simulink model "LOPES_3D"  (R2015b)
settings: Solver=ode3  StartTime=0.0  StopTime=inf  FixedStep=ts  RelTol=1e-3
PostLoadFcn:
  | DataFileTemplate = 'd:\%d_LNMC_S01_SLRT_%i.mat';
InitFcn:
  | cd(fileparts(which(gcs)));
  | runScripts
StartFcn:
  | cd(fileparts(which(gcs)));
StopFcn:
  | SaveSLRTData(DataFileTemplate)
values from neighbouring files (symbols this model uses):
  SelectorLOPESInSize = 8    [setAnkleDepInd.m]
libraries: nmc x51, simulink x22, slrtlib x14, LopesDevelopmentLibrary x7, dspsigops x1
(part 1 of 2)
settings Model: xpc_rtwmakecfg_data=_xpciplib__xpcnblib__xpcetherlib__xpcether8255xlib__xpcetherGbElib_  SimulationMode=external  Creator=OortG  LastModifiedBy=brugtjh
settings SolverCC: EnableConcurrentExecution=on
settings DataIOCC: SaveFormat=Array
settings OptimizationCC: BlockReduction=off  OptimizeBlockIOStorage=off  BufferReuse=off  GlobalBufferReuse=off  ExpressionFolding=off  ExpressionDepthLimit=2147483647  LocalBlockOutputs=off
settings DebuggingCC: UnderspecifiedInitializationDetection=Classic  MergeDetectMultiDrivingBlocksExec=none  SolverPrmCheckMsg=warning  StateNameClashWarn=warning
settings HardwareCC: ProdBitPerPointer=32  ProdLargestAtomicFloat=None  ProdWordSize=32  ProdLongLongMode=on  ProdHWDeviceType=Generic->32-bit x86 compatible
settings RTWCC: SystemTargetFile=slrt.tlc  TLCOptions=-axPCMaxOverloads=999999 -axPCOverLoadLen=999999 -axPCStartupFlag=5  TemplateMakefile=slrt_default_tmf  Description=Simulink Real-Time
settings ConfigComp: CovModelRefEnable=Off

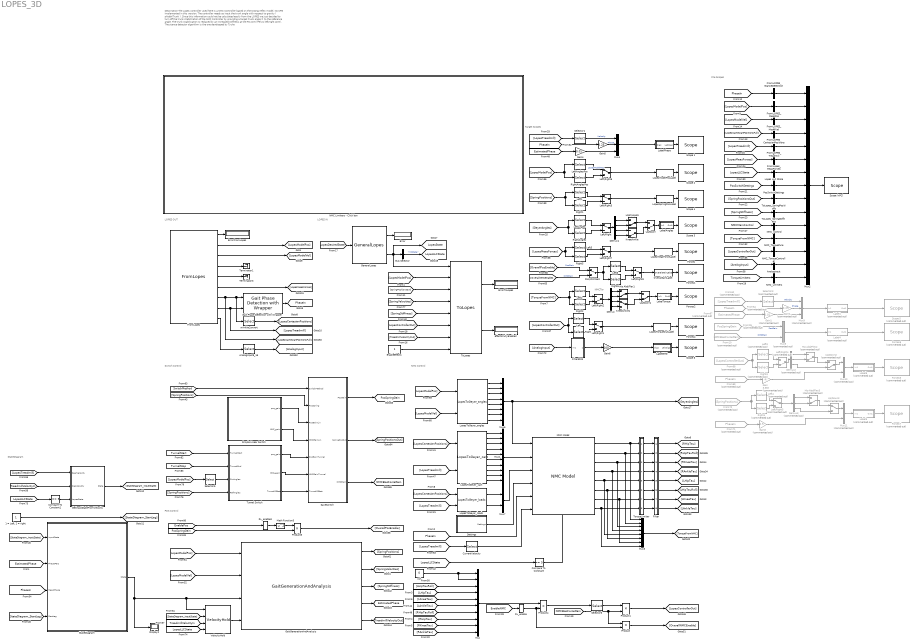
== system LOPES_3D ==
  note: File Scopes
  note: Description
      |
      | The Lopes controller used here is a NMC Controller based on the S.Song reflex model. No CPG Implemented in this version.
      |
      | The controller needs as input the trunk angle with respect to gravity ( phidphiTrunk ).
      | Since this information could not be calculated easily from the LOPES we just decided to turn off the trunk stabilization of the NMC Controller by providing a target trunk angle = to the reference angle.
      |
      | The trunk stabilization is replaced by an increased stiffness at the PZ joint (Pelvis left/right joint).
      |
      | The stance detector algorithm is the one developped by Tycho
  note: Target Scopes
  note: LOPES OUT
  note: LOPES IN
  note: NMC Control
  note: NMCTor
  note: Switch Control
  note: POS Control
  note: StateDiagram
  "1 = Left, 2 = right" : Constant
  AnalogInput : Concatenate  NumInputs=1
  AnalogInput9_16 : Selector  InputPortWidth=16  IndexOptions=Index vector (dialog)  Indices=9:16  OutputSizes=1
  Bus Selector : BusSelector  OutputSignals=llcState
  Compare To Constant : simulink/Logic and Bit Operations/Compare To Constant  relop===  const=5  OutDataTypeStr=boolean
  Compare To Constant1 : simulink/Logic and Bit Operations/Compare To Constant  relop===  const=5  OutDataTypeStr=boolean
  CurrentVelocity : Selector  InputPortWidth=7  IndexOptions=Index vector (dialog)  Indices=[2]  OutputSizes=1
  Demux : Demux
  Demux1 : Demux
  Demux2 : Demux  Commented=on  Outputs=3
  Demux3 : Demux  Commented=on  Outputs=3
  Display2 : Display
  EffectsFullyEnabled : Display
      settings: AttributesFormatString=%<Tag>
  EnableEffects : Constant  OutDataTypeStr=double
      settings: OpenFcn=|
      | b = get_param(gcb,'value');
      | if (strcmp(b,'1')),
      |   set_param (gcb,'value','0');
      | else
      |   set_param(gcb,'value','1');
      | end;
  Error : Display
      settings: AttributesFormatString=%<Tag>
  ErrorFromLopes : Display
      settings: AttributesFormatString=%<Tag>
  ErrorToLopes : Display
      settings: AttributesFormatString=%<Tag>
  Filter : Subsystem
  FilterEMG : Subsystem
  Forces : slrtlib/Displays and Logging/Scope   scopeno=6  scopetype=Target  autostart=on  viewmode=Graphical sliding  formatstr='%15.6f'  grid=on  ylimits=[0,0]  nosamples=5000  noprepostsamples=0  interleave=1  triggermode=FreeRun  triggersignal=1  trigsignalfromport=off  triggerlevel=0.0  triggerslope=Either  triggerscope=1  triggersample=0  filename=data.dat  mode=Lazy  writesize=512  autorestart=off  dynamicfilemode=off  maxwritefilesize=512*1024^2
  Forces1 : slrtlib/Displays and Logging/Scope   scopeno=7  scopetype=Target  autostart=on  viewmode=Graphical sliding  formatstr='%15.6f'  grid=on  ylimits=[0,0]  nosamples=5000  noprepostsamples=0  interleave=1  triggermode=FreeRun  triggersignal=1  trigsignalfromport=off  triggerlevel=0.0  triggerslope=Either  triggerscope=1  triggersample=0  filename=data.dat  mode=Lazy  writesize=512  autorestart=off  dynamicfilemode=off  maxwritefilesize=512*1024^2
  Forces2 : slrtlib/Displays and Logging/Scope   scopeno=8  scopetype=Target  autostart=on  viewmode=Graphical sliding  formatstr='%15.6f'  grid=on  ylimits=[0,0]  nosamples=5000  noprepostsamples=0  interleave=1  triggermode=FreeRun  triggersignal=1  trigsignalfromport=off  triggerlevel=0.0  triggerslope=Either  triggerscope=1  triggersample=0  filename=data.dat  mode=Lazy  writesize=512  autorestart=off  dynamicfilemode=off  maxwritefilesize=512*1024^2
  Forces4 : slrtlib/Displays and Logging/Scope   scopeno=9  scopetype=Target  autostart=on  viewmode=Graphical sliding  formatstr='%15.6f'  grid=on  ylimits=[0,0]  nosamples=5000  noprepostsamples=0  interleave=1  triggermode=FreeRun  triggersignal=1  trigsignalfromport=off  triggerlevel=0.0  triggerslope=Either  triggerscope=1  triggersample=0  filename=data.dat  mode=Lazy  writesize=512  autorestart=off  dynamicfilemode=off  maxwritefilesize=512*1024^2
  Forces5 : slrtlib/Displays and Logging/Scope   Commented=on  scopeno=33  scopetype=Target  autostart=on  viewmode=Graphical sliding  formatstr='%15.6f'  grid=on  ylimits=[-20,20]  nosamples=5000  noprepostsamples=0  interleave=1  triggermode=FreeRun  triggersignal=1  trigsignalfromport=off  triggerlevel=0.0  triggerslope=Either  triggerscope=1  triggersample=0  filename=data.dat  mode=Lazy  writesize=512  autorestart=off  dynamicfilemode=off  maxwritefilesize=512*1024^2
  Forces6 : slrtlib/Displays and Logging/Scope   Commented=on  scopeno=22  scopetype=Target  autostart=on  viewmode=Graphical sliding  formatstr='%15.6f'  grid=on  ylimits=[0,0]  nosamples=5000  noprepostsamples=0  interleave=1  triggermode=FreeRun  triggersignal=1  trigsignalfromport=off  triggerlevel=0.0  triggerslope=Either  triggerscope=1  triggersample=0  filename=data.dat  mode=Lazy  writesize=512  autorestart=off  dynamicfilemode=off  maxwritefilesize=512*1024^2
  Forces7 : slrtlib/Displays and Logging/Scope   Commented=on  scopeno=44  scopetype=Target  autostart=on  viewmode=Graphical sliding  formatstr='%15.6f'  grid=on  ylimits=[-3,3]  nosamples=5000  noprepostsamples=0  interleave=1  triggermode=FreeRun  triggersignal=1  trigsignalfromport=off  triggerlevel=0.0  triggerslope=Either  triggerscope=1  triggersample=0  filename=data.dat  mode=Lazy  writesize=512  autorestart=off  dynamicfilemode=off  maxwritefilesize=512*1024^2
  From10 : From  Commented=on  GotoTag=NMCBiasForceGain  TagVisibility=global
  From26 : From  Commented=on  GotoTag=PosSpringGain  TagVisibility=global
  From62 : From  Commented=on  GotoTag=LopesTreadmill
  From64 : From  Commented=on  GotoTag=PhaseIn  TagVisibility=global
  From67 : From  Commented=on  GotoTag=EstimatedPhase  TagVisibility=global
  From68 : From  Commented=on  GotoTag=LopesControllerOut
  From69 : From  Commented=on  GotoTag=PhaseIn  TagVisibility=global
  From70 : From  Commented=on  GotoTag=SpringPositions
  From71 : From  Commented=on  GotoTag=PhaseIn  TagVisibility=global
  FromLOPES_CartesianPositions : Concatenate  NumInputs=1
  FromLOPES_MeasPos : Concatenate  NumInputs=1
  FromLOPES_ModelVel : Concatenate  NumInputs=1
  FromLOPES_StanceDetection : Concatenate  NumInputs=1
  FromLOPES_Treadmill : Concatenate  NumInputs=1
  FromLopes : LopesDevelopmentLibrary/Robot control blocks/FromLopes
  FromLopes_MeasForces : Concatenate  NumInputs=1
  Gain : Gain  Commented=on  Gain=3.333
  Gain1 : Gain  Commented=on  Gain=0.01
  Gain2 : Gain  Commented=on  Gain=0.25
  Gain3 : Gain  Commented=on  Gain=0.5
  Gain4 : Gain  Gain=0.01
  Gain5 : Gain  Gain=0.25
  Gain6 : Gain  Gain=100
  Gait Phase Detection with Wrapper : LopesDevelopmentLibrary/GaitPhaseDetection/Gait Phase Detection with Wrapper
  GaitGenerationAndAnalysis : LopesDevelopmentLibrary/GaitGenerationExtra/GaitGenerationAndAnalysis
      link override "CalculateBreaksCoefs/Calculate/StartLeft ": SetVelocity=0.1
      link override CalculateBreaksCoefs/Calculate/StartRight: SetVelocity=0.1
      link override CalculateBreaksCoefs/Calculate/StopLeft: SetVelocity=0.3
      link override CalculateBreaksCoefs/Calculate/StopRight: SetVelocity=0.3
      link override PhaseEstimatorAoyagi_wPI_Extra: AoyagiFilterGain=2
  GeneralLopes : LopesDevelopmentLibrary/Robot control blocks/GeneralLopes
  GetInputStateFromVelocity : Subsystem
  Hip Abd/Flex1 : ManualSwitch  CurrentSetting=0
  Hip Abd/Flex2 : ManualSwitch  Commented=on  CurrentSetting=0
  Hip Abd/Flex3 : ManualSwitch  Commented=on  CurrentSetting=0
  HipFl/HipAb : ManualSwitch  CurrentSetting=0
  Knee/Ankle : ManualSwitch  CurrentSetting=0
  Knee/Ankle1 : ManualSwitch
  Label1 : Subsystem  Commented=on
  Label4 : Subsystem  Commented=on
  Label5 : Subsystem  Commented=on
  Label6 : Subsystem  Commented=on
  LabelAngles : Subsystem
  LabelEMG : Subsystem
  LabelPhase : Subsystem
  LabelTorque : Subsystem
  Left{,1,5..6} (4 alike) : Selector  InputPortWidth=SelectorScopesSize  IndexOptions=Index vector (dialog)  Indices=SelectorScopesLeft  OutputSizes=1
  Left/Right{,1,3,6..7} (5 alike) : ManualSwitch
  Left/Right2 : ManualSwitch  CurrentSetting=0
  Left/Right4 : ManualSwitch  Commented=on  CurrentSetting=0
  Left/Right5 : ManualSwitch  Commented=on
  "Left/Right8 " : ManualSwitch
  Left2 : Selector  InputPortWidth=8  IndexOptions=Index vector (dialog)  Indices=[5,6,7,8]  OutputSizes=1
  Left3 : Selector  Commented=on  InputPortWidth=SelectorScopesSize  IndexOptions=Index vector (dialog)  Indices=SelectorScopesLeft  OutputSizes=1
  Left4 : Selector  Commented=on  InputPortWidth=SelectorScopesSize  IndexOptions=Index vector (dialog)  Indices=SelectorScopesLeft  OutputSizes=1
  LeftAngles : Selector  InputPortWidth=16  IndexOptions=Index vector (dialog)  Indices=[1,3,5,7]  OutputSizes=1
  LeftAnglesPos : Selector  InputPortWidth=SelectorLOPESModelPosSize  IndexOptions=Index vector (dialog)  Indices=SelectorScopesLeft  OutputSizes=1
  Lopes LLC State : Concatenate  NumInputs=1
  LopesMeasForceLabel : nmc/LopesMeasForceLabel
  LopesModelPosLabel : nmc/LopesModelPosLabel
  LopesSpringPosLabel : nmc/LopesSpringPosLabel
  LopesToGeyer_angles : nmc/LopesToGeyer_angles
  LopesToGeyer_cart : nmc/LopesToGeyer_cart
  LopesToGeyer_loads : nmc/LopesToGeyer_loads
  LopesTorqueOutLabel : nmc/LopesTorqueOutLabel
  Math Function3 : Math  Operator=square  SaturateOnIntegerOverflow=on
  Mux : Mux  Inputs=10
  Mux1 : Mux  Inputs=10
  Mux10 : Mux  Commented=on  Inputs=2
  Mux11 : Mux  Commented=on  Inputs=2
  Mux2 : Mux  Inputs=15
  Mux3 : Mux  Inputs=8
  Mux4 : Mux  Inputs=3
  Mux5 : Mux  Commented=on  Inputs=2
  Mux6 : Mux  Inputs=8
  Mux7 : Mux  Inputs=2
  Mux9 : Mux  Commented=on  Inputs=3
  NMC Limiters - Click box : Subsystem  mask{LopesDesiredState=Init, VelocityTreadmill=1, PercLimiterRate=20, InfoShow_LLC=0, InfoShow_Blue=1, InfoShow_Init=0, InfoShow_Motors=0, InfoShow_Treadmill=0, InfoShow_Patient=1, EnablePos=Enable, PosControlType=Linear, PosLimiterPercentageSymmetric=0.0, PosLimiterPercentagePelvis=0.0, PosLimiterPercentageLeft=8.0, PosLimiterPercentageRight=0.0, DisableAddPelvis=off, DisableAddLeft=off, DisableAddRight=off, Pos_Tunnel_PelvisX=0.010, Pos_Tunnel_PelvisZ=0.010, Pos_Tunnel_HipAdd=0.100, Pos_Tunnel_PelvisX_Out=0.020, Pos_Tunnel_PelvisZ_Out=0.020, Pos_Tunnel_HipAdd_Out=0.200, Pos_Tunnel_HipFlx=0.100, Pos_Tunnel_Knee=0.100, Pos_Tunnel_Ankle=0.200, Pos_Tunnel_HipFlx_Out=0.200, Pos_Tunnel_Knee_Out=0.200, Pos_Tunnel_Ankle_Out=0.400, EnableNMC=Enable, TorqueLimiterPercentageSymmetric=0, TorqueLimiterPercentageLeft=0, TorqueLimiterPercentageRight=0, GradientFunctionSwitch=Per Gradient, NMC_HipAddAbd_Percentage=100.0, NMC_HipFlexExt_Percentage=100, NMC_KneeFlexExt_Percentage=0, NMC_AnkleDorsPlant_Percentage=0, NMC_HipAdd_Percentage=100.0, NMC_HipAbd_Percentage=100.0, NMC_HipFlexors_Percentage=100, NMC_HipExtensors_Percentage=100, NMC_KneeFlexors_Percentage=0, NMC_KneeExtensors_Percentage=100, NMC_AnkleDFlexor_Percentage=0, NMC_AnklePFlexors_Percentage=0, NMC_HipMuscles_AbAd_Percentage=100.0, NMC_HipMuscles_FE_Percentage=100.0, NMC_BiArticularMuscles_HK_Percentage=100.0, NMC_KneeMuscles_Percentage=100.0, NMC_BiArticularMuscles_KA_Percentage=0.0, NMC_AnkleMuscles_Percentage=0.0, EnableJointLimits=Disable, UseConstantPitch=Enable, UsePredictedAnkle=Enable, KneeAngleBias=0, FilterFreq=25, EnableStandingStill=Enable, StandingStillLimitFront=0.10, StandingStillLimitSide=0.20}
      mask prompts: LopesDesiredState "Lopes State (Desired):"; VelocityTreadmill "Treadmill Velocity (m/s):"; PercLimiterRate "Limiter Rate (%/s):"; InfoShow_LLC "LLC State"; InfoShow_Blue "Blue Cabinet Pressed"; InfoShow_Init "Init OK"; InfoShow_Motors "Motors OK"; InfoShow_Treadmill "Treadmill Empty"; InfoShow_Patient "PatientDefined"; EnablePos "Enable/Disable Pos"; PosLimiterPercentageSymmetric "Overal Gain:"; PosLimiterPercentagePelvis "Pelvis Gain:"; PosLimiterPercentageLeft "Left Gain:"; PosLimiterPercentageRight "Right Gain:"; DisableAddPelvis "Disable Tunnel Pelvis"; DisableAddLeft "Disable Tunnel Left"; DisableAddRight "Disable Tunnel Right"; Pos_Tunnel_PelvisX "Pelvis (x) (m):"; Pos_Tunnel_PelvisZ "Pelvis (z) (m):"; Pos_Tunnel_HipAdd "Hip Add/Abd (rad):"; Pos_Tunnel_PelvisX_Out "Pelvis (x) (m):"; Pos_Tunnel_PelvisZ_Out "Pelvis (z) (m):"; Pos_Tunnel_HipAdd_Out "Hip Add/Abd (rad):"; Pos_Tunnel_HipFlx "Hip Flx/Ext (rad):"; Pos_Tunnel_Knee "Knee Flx/Ext (rad):"; Pos_Tunnel_Ankle "Ankle Flx/Ext (rad):"; Pos_Tunnel_HipFlx_Out "Hip Flx/Ext (rad):"; Pos_Tunnel_Knee_Out "Knee Flx/Ext (rad):"; Pos_Tunnel_Ankle_Out "Ankle Flx/Ext (rad):"; EnableNMC "Enable/Disable NMC"; TorqueLimiterPercentageSymmetric "Overal Gain:"; TorqueLimiterPercentageLeft "Left Gain:"; TorqueLimiterPercentageRight "Right Gain:"; NMC_HipAddAbd_Percentage "Hip Add/Abd Percentage"; NMC_HipFlexExt_Percentage "Hip Flex/Ext Percentage"; NMC_KneeFlexExt_Percentage "Knee Flex/Ext Percentage"; NMC_AnkleDorsPlant_Percentage "Ankle Dorsi/Plantar Percentage"; NMC_HipAdd_Percentage "Hip Adduction Percentage"; NMC_HipAbd_Percentage "Hip Abduction Percentage"; NMC_HipFlexors_Percentage "Hip Flexor Percentage"; NMC_HipExtensors_Percentage "Hip Extensor Percentage"; NMC_KneeFlexors_Percentage "Knee Flexor Percentage"; NMC_KneeExtensors_Percentage "Knee Extensor Percentage"; NMC_AnkleDFlexor_Percentage "Ankle DorsiFlexor Percentage"; NMC_AnklePFlexors_Percentage "Ankle PlantarFlexor Percentage"; NMC_HipMuscles_AbAd_Percentage "Hip (Mono) (Abd/Add)"; NMC_HipMuscles_FE_Percentage "Hip (Mono) (Flex./Ext.)"; NMC_BiArticularMuscles_HK_Percentage "Hip/Knee (BiArt)"; NMC_KneeMuscles_Percentage "Knee (Mono)"; NMC_BiArticularMuscles_KA_Percentage "Knee/Ankle (BiArt)"; NMC_AnkleMuscles_Percentage "Ankle Muscles"; EnableJointLimits "Enable/Disable Joint Limits"; UseConstantPitch "Enable/Disable Constant Pitch"; UsePredictedAnkle "Enable/Disable Predicted Ankle"; KneeAngleBias "Knee Angle Bias (Rad):"; FilterFreq "Filter Frequency (Hz):"; EnableStandingStill "Enable/Disable Standing Still"; StandingStillLimitFront "Front Velocity Limit"; StandingStillLimitSide "Side Velocity Limit"
      mask TypeOptions LopesDesiredState: Off | Init | Force
      mask Callback LopesDesiredState:
      | button_value = get_param(gcb,'LopesDesiredState');
      | 
      | if strcmp(button_value,'Off')
      |      set_param([gcb '/DesiredState'],'Value',num2str(0));
      | elseif strcmp(button_value,'Init')
      |     set_param([gcb '/DesiredState'],'Value',num2str(1));
      | elseif strcmp(button_value,'Force')
      |     set_param([gcb '/DesiredState'],'Value',num2str(5));
      | end
      mask Callback PercLimiterRate:
      | button_value = get_param(gcb,'PercLimiterRate');
      | set_param([gcb '/PercLimiterRate'],'Value',num2str(button_value));
      mask TypeOptions EnablePos: Enable | Disable
      mask Callback EnablePos:
      | button_value = get_param(gcb,'EnablePos');
      | 
      | if strcmp(button_value,'Enable')
      |      set_param([gcb '/EnablePos'],'Value',num2str(1));
      |      set_param([gcb '/DisableAddAll'],'Value','0');
      | else
      |     set_param([gcb '/EnablePos'],'Value',num2str(0));
      |     set_param([gcb '/DisableAddAll'],'Value','2*pi');
      | end
      mask TypeOptions PosControlType: Linear | Tunnel
      mask Callback PosControlType:
      | button_value = get_param(gcb,'PosControlType');
      | 
      | maskHandle = Simulink.Mask.get(gcb);
      | buttonHandleTunnel1 = maskHandle.getDialogControl('ContainerTunnel1');
      | buttonHandleTunnel2 = maskHandle.getDialogControl('ContainerTunnel2');
      | % buttonHandleDisableTunnelPelvis = maskHandle.getParameter('DisableAddPelvis');
      | % buttonHandleDisableTunnelLeft = maskHandle.getParameter('DisableAddLeft');
      | % buttonHandleDisableTunnelRight = maskHandle.getParameter('DisableAddRight');
      | if strcmp(button_value,'Tunnel')
      |     set_param([gcb '/PosControlType'],'Value',num2str(1));
      |     buttonHandleTunnel1.Enabled = 'on';
      |     buttonHandleTunnel2.Enabled = 'on';
      | %     buttonHandleDisableTunnelPelvis.Enabled = 'on';
      | %     buttonHandleDisableTunnelLeft.Enabled = 'on';
      | %     buttonHandleDisableTunnelRight.Enabled = 'on';
      | else
      |     set_param([gcb '/PosControlType'],'Value',num2str(0));
      |     buttonHandleTunnel1.Enabled = 'off';
      |     buttonHandleTunnel2.Enabled = 'off';
      | %     buttonHandleDisableTunnelPelvis.Enabled = 'off';
      | %     buttonHandleDisableTunnelLeft.Enabled = 'off';
      | %     buttonHandleDisableTunnelRight.Enabled = 'off';
      | end
      mask Callback PosLimiterPercentageSymmetric:
      | %% Overal Gain
      | value_new = get_param(gcb,'PosLimiterPercentageSymmetric');
      | value = get_param([gcb,'/PosLimiterPercentage'],'Value');
      | 
      | if ~strcmp(value,value_new)
      | % Also setting other sliders
      | set_param(gcb,'PosLimiterPercentagePelvis',value_new);
      | set_param(gcb,'PosLimiterPercentageLeft',value_new);
      | set_param(gcb,'PosLimiterPercentageRight',value_new);
      | 
      | % Setting Overal Slider (Only used for logging)
      | set_param([gcb '/PosLimiterPercentage'],'Value',value_new);
      | end
      mask Callback DisableAddPelvis:
      | value = get_param(gcb,'DisableAddPelvis');
      | 
      | if strcmp(value,'on')
      |     set_param([gcb,'/DisableAddPelvis'],'Value','2*pi')
      | else
      | set_param([gcb,'/DisableAddPelvis'],'Value','0')
      | end
      mask Callback DisableAddLeft:
      | value = get_param(gcb,'DisableAddLeft');
      | 
      | if strcmp(value,'on')
      |     set_param([gcb,'/DisableAddLeft'],'Value','2*pi')
      | else
      | set_param([gcb,'/DisableAddLeft'],'Value','0')
      | end
      mask Callback DisableAddRight:
      | value = get_param(gcb,'DisableAddRight');
      | 
      | if strcmp(value,'on')
      |     set_param([gcb,'/DisableAddRight'],'Value','2*pi')
      | else
      |     set_param([gcb,'/DisableAddRight'],'Value','0')
      | end
      mask Callback Pos_Tunnel_PelvisX:
      | %% Overal Gain
      | value_first = get_param(gcb,'Pos_Tunnel_PelvisX');
      | value = get_param(gcb,'Pos_Tunnel_PelvisX_Out');
      | 
      | if str2num(value) < str2num(value_first)
      |     set_param(gcb,'Pos_Tunnel_PelvisX_Out',value_first);
      | end
      mask Callback Pos_Tunnel_PelvisZ:
      | %% Overal Gain
      | value_first = get_param(gcb,'Pos_Tunnel_PelvisZ');
      | value = get_param(gcb,'Pos_Tunnel_PelvisZ_Out');
      | 
      | if str2num(value) < str2num(value_first)
      |     set_param(gcb,'Pos_Tunnel_PelvisZ_Out',value_first);
      | end
      mask Callback Pos_Tunnel_HipAdd:
      | %% Overal Gain
      | value_first = get_param(gcb,'Pos_Tunnel_HipAdd');
      | value = get_param(gcb,'Pos_Tunnel_HipAdd_Out');
      | 
      | if str2num(value) < str2num(value_first)
      |     set_param(gcb,'Pos_Tunnel_HipAdd_Out',value_first);
      | end
      mask Callback Pos_Tunnel_PelvisX_Out:
      | %% Overal Gain
      | value = get_param(gcb,'Pos_Tunnel_PelvisX_Out');
      | value_first = get_param(gcb,'Pos_Tunnel_PelvisX');
      | 
      | if str2num(value) < str2num(value_first)
      |     set_param(gcb,'Pos_Tunnel_PelvisX_Out',value_first);
      | end
      mask Callback Pos_Tunnel_PelvisZ_Out:
      | %% Overal Gain
      | value = get_param(gcb,'Pos_Tunnel_PelvisZ_Out');
      | value_first = get_param(gcb,'Pos_Tunnel_PelvisZ');
      | 
      | if str2num(value) < str2num(value_first)
      |     set_param(gcb,'Pos_Tunnel_PelvisZ_Out',value_first);
      | end
      mask Callback Pos_Tunnel_HipAdd_Out:
      | %% Overal Gain
      | value = get_param(gcb,'Pos_Tunnel_HipAdd_Out');
      | value_first = get_param(gcb,'Pos_Tunnel_HipAdd');
      | 
      | if str2num(value) < str2num(value_first)
      |     set_param(gcb,'Pos_Tunnel_HipAdd_Out',value_first);
      | end
      mask Callback Pos_Tunnel_HipFlx:
      | %% Overal Gain
      | value_first = get_param(gcb,'Pos_Tunnel_HipFlx');
      | value = get_param(gcb,'Pos_Tunnel_HipFlx_Out');
      | 
      | if str2num(value) < str2num(value_first)
      |     set_param(gcb,'Pos_Tunnel_HipFlx_Out',value_first);
      | end
      mask Callback Pos_Tunnel_Knee:
      | %% Overal Gain
      | value_first = get_param(gcb,'Pos_Tunnel_Knee');
      | value = get_param(gcb,'Pos_Tunnel_Knee_Out');
      | 
      | if str2num(value) < str2num(value_first)
      |     set_param(gcb,'Pos_Tunnel_Knee_Out',value_first);
      | end
      mask Callback Pos_Tunnel_Ankle:
      | %% Overal Gain
      | value_first = get_param(gcb,'Pos_Tunnel_Ankle');
      | value = get_param(gcb,'Pos_Tunnel_Ankle_Out');
      | 
      | if str2num(value) < str2num(value_first)
      |     set_param(gcb,'Pos_Tunnel_Ankle_Out',value_first);
      | end
      mask Callback Pos_Tunnel_HipFlx_Out:
      | %% Overal Gain
      | value = get_param(gcb,'Pos_Tunnel_HipFlx_Out');
      | value_first = get_param(gcb,'Pos_Tunnel_HipFlx');
      | 
      | if str2num(value) < str2num(value_first)
      |     set_param(gcb,'Pos_Tunnel_HipFlx_Out',value_first);
      | end
      mask Callback Pos_Tunnel_Knee_Out:
      | %% Overal Gain
      | value = get_param(gcb,'Pos_Tunnel_Knee_Out');
      | value_first = get_param(gcb,'Pos_Tunnel_Knee');
      | 
      | if str2num(value) < str2num(value_first)
      |     set_param(gcb,'Pos_Tunnel_Knee_Out',value_first);
      | end
      mask Callback Pos_Tunnel_Ankle_Out:
      | %% Overal Gain
      | value = get_param(gcb,'Pos_Tunnel_Ankle_Out');
      | value_first = get_param(gcb,'Pos_Tunnel_Ankle');
      | 
      | if str2num(value) < str2num(value_first)
      |     set_param(gcb,'Pos_Tunnel_Ankle_Out',value_first);
      | end
      mask TypeOptions EnableNMC: Enable | Disable
      mask Callback EnableNMC:
      | button_value = get_param(gcb,'EnableNMC');
      | 
      | if strcmp(button_value,'Enable')
      |      set_param([gcb '/EnableNMC'],'Value',num2str(1));
      | else
      |     set_param([gcb '/EnableNMC'],'Value',num2str(0));
      | end
      mask Callback TorqueLimiterPercentageSymmetric:
      | %% Overal Gain
      | value_new = get_param(gcb,'TorqueLimiterPercentageSymmetric');
      | value = get_param([gcb,'/TorqueLimiterPercentageSymmetric'],'Value');
      | 
      | if ~strcmp(value,value_new)
      | % Also setting other sliders
      | set_param(gcb,'TorqueLimiterPercentageLeft',value_new);
      | set_param(gcb,'TorqueLimiterPercentageRight',value_new);
      | 
      | % Setting Overal Slider (Only used for logging)
      | set_param([gcb '/TorqueLimiterPercentageSymmetric'],'Value',value_new);
      | end
      mask TypeOptions GradientFunctionSwitch: Per Joint | Per Function | Per Gradient
      mask Callback GradientFunctionSwitch:
      | blk = gcb;
      | button_value = get_param(gcb,'GradientFunctionSwitch');
      | 
      | if strcmp(button_value,'Per Joint')
      |     DesiredControlMethod = 1;
      | elseif strcmp(button_value,'Per Function')
      |     DesiredControlMethod = 2;
      | elseif strcmp(button_value,'Per Gradient')
      |     DesiredControlMethod = 3;
      | end
      | 
      | set_param([gcb '/LimiterMethod'],'Value',num2str(DesiredControlMethod));
      | 
      | %% Disabling one or the other
      | maskHandle = Simulink.Mask.get(gcb);
      | buttonHandleGradient = maskHandle.getDialogControl('Container_Gradient');
      | buttonHandleFunction = maskHandle.getDialogControl('Container_Function');
      | buttonHandleJoint = maskHandle.getDialogControl('Container_Joint');
      | if DesiredControlMethod == 1 %Per Joint
      |     buttonHandleGradient.Enabled = 'off';
      |     buttonHandleFunction.Enabled = 'off';
      |     buttonHandleJoint.Enabled = 'on';
      | elseif DesiredControlMethod == 2 %Per Function
      |     buttonHandleGradient.Enabled = 'off';
      |     buttonHandleFunction.Enabled = 'on';
      |     buttonHandleJoint.Enabled = 'off';
      | elseif DesiredControlMethod == 3 %Per Gradient
      |     buttonHandleGradient.Enabled = 'on';
      |     buttonHandleFunction.Enabled = 'off';
      |     buttonHandleJoint.Enabled = 'off';
      | end
      mask Callback NMC_HipAddAbd_Percentage:
      | %Setting values hip add/abd
      | if str2num(get_param([gcb '/LimiterMethod'],'Value')) == 1;
      |     %Also setting values of sliders per joint/per location
      |     set_param(gcb,'NMC_HipAdd_Percentage',get_param(gcb,'NMC_HipAddAbd_Percentage'))
      |     set_param(gcb,'NMC_HipAbd_Percentage',get_param(gcb,'NMC_HipAddAbd_Percentage'))
      |     set_param(gcb,'NMC_HipMuscles_AbAd_Percentage',get_param(gcb,'NMC_HipAddAbd_Percentage'))
      | end
      mask Callback NMC_HipFlexExt_Percentage:
      | if str2num(get_param([gcb '/LimiterMethod'],'Value')) == 1;
      | %Also setting values of sliders per function/per location
      | %Per Function
      | set_param(gcb,'NMC_HipFlexors_Percentage',str2num(get_param(gcb,'NMC_HipFlexExt_Percentage')))
      | set_param(gcb,'NMC_HipExtensors_Percentage',str2num(get_param(gcb,'NMC_HipFlexExt_Percentage')))
      | 
      | %Per Location
      | set_param(gcb,'NMC_HipMuscles_FE_Percentage',str2num(get_param(gcb,'NMC_HipFlexExt_Percentage')))
      | set_param(gcb,'NMC_BiArticularMuscles_HK_Percentage',min([str2num(get_param(gcb,'NMC_HipFlexExt_Percentage')) str2num(get_param(gcb,'NMC_KneeFlexExt_Percentage'))]))
      | end
      mask Callback NMC_KneeFlexExt_Percentage:
      | if str2num(get_param([gcb '/LimiterMethod'],'Value')) == 1;
      | %Also setting values of sliders per joint/per location
      | set_param(gcb,'NMC_KneeFlexors_Percentage',str2num(get_param(gcb,'NMC_KneeFlexExt_Percentage')))
      | set_param(gcb,'NMC_KneeExtensors_Percentage',str2num(get_param(gcb,'NMC_KneeFlexExt_Percentage')))
      | set_param(gcb,'NMC_KneeMuscles_Percentage',str2num(get_param(gcb,'NMC_KneeFlexExt_Percentage')))
      | set_param(gcb,'NMC_BiArticularMuscles_KA_Percentage',min([str2num(get_param(gcb,'NMC_KneeFlexExt_Percentage')) str2num(get_param(gcb,'NMC_AnkleDorsPlant_Percentage'))]))
      | set_param(gcb,'NMC_BiArticularMuscles_HK_Percentage',min([str2num(get_param(gcb,'NMC_HipFlexExt_Percentage')) str2num(get_param(gcb,'NMC_KneeFlexExt_Percentage'))]))
      | end
      mask Callback NMC_AnkleDorsPlant_Percentage:
      | if str2num(get_param([gcb '/LimiterMethod'],'Value')) == 1;
      | %Also setting values of sliders per joint/per location
      | set_param(gcb,'NMC_AnkleDFlexor_Percentage',str2num(get_param(gcb,'NMC_AnkleDorsPlant_Percentage')))
      | set_param(gcb,'NMC_AnklePFlexors_Percentage',str2num(get_param(gcb,'NMC_AnkleDorsPlant_Percentage')))
      | set_param(gcb,'NMC_AnkleMuscles_Percentage',str2num(get_param(gcb,'NMC_AnkleDorsPlant_Percentage')))
      | set_param(gcb,'NMC_BiArticularMuscles_KA_Percentage',min([str2num(get_param(gcb,'NMC_KneeFlexExt_Percentage')) str2num(get_param(gcb,'NMC_AnkleDorsPlant_Percentage'))]))
      | end
      mask Callback NMC_HipAdd_Percentage:
      | if str2num(get_param([gcb '/LimiterMethod'],'Value')) == 2;
      | %Also setting values of sliders per joint/per location
      | set_param(gcb,'NMC_HipAddAbd_Percentage',min([str2num(get_param(gcb,'NMC_HipAdd_Percentage')) str2num(get_param(gcb,'NMC_HipAbd_Percentage'))]))
      | set_param(gcb,'NMC_HipMuscles_AbAd_Percentage',min([str2num(get_param(gcb,'NMC_HipAdd_Percentage')) str2num(get_param(gcb,'NMC_HipAbd_Percentage'))]))
      | end
      mask Callback NMC_HipAbd_Percentage:
      | if str2num(get_param([gcb '/LimiterMethod'],'Value')) == 2;
      | %Also setting values of sliders per joint/per location
      | set_param(gcb,'NMC_HipAddAbd_Percentage',min([str2num(get_param(gcb,'NMC_HipAdd_Percentage')) str2num(get_param(gcb,'NMC_HipAbd_Percentage'))]))
      | set_param(gcb,'NMC_HipMuscles_AbAd_Percentage',min([str2num(get_param(gcb,'NMC_HipAdd_Percentage')) str2num(get_param(gcb,'NMC_HipAbd_Percentage'))]))
      | end
      mask Callback NMC_HipFlexors_Percentage:
      | if str2num(get_param([gcb '/LimiterMethod'],'Value')) == 2;
      | 
      | %% Also setting values of sliders per joint/per location
      | % Per Joint
      | set_param(gcb,'NMC_HipFlexExt_Percentage',min([str2num(get_param(gcb,'NMC_HipFlexors_Percentage')) str2num(get_param(gcb,'NMC_HipExtensors_Percentage'))]))
      | 
      | % Per Location
      | set_param(gcb,'NMC_HipMuscles_FE_Percentage',min([str2num(get_param(gcb,'NMC_HipFlexors_Percentage')) str2num(get_param(gcb,'NMC_HipExtensors_Percentage'))]))
      | set_param(gcb,'NMC_BiArticularMuscles_HK_Percentage',min([str2num(get_param(gcb,'NMC_KneeExtensors_Percentage')) str2num(get_param(gcb,'NMC_KneeFlexors_Percentage')) str2num(get_param(gcb,'NMC_HipFlexors_Percentage')) str2num(get_param(gcb,'NMC_HipExtensors_Percentage'))]))
      | end
      mask Callback NMC_HipExtensors_Percentage:
      | if str2num(get_param([gcb '/LimiterMethod'],'Value')) == 2;
      | %Also setting values of sliders per joint/per location
      | set_param(gcb,'NMC_HipFlexExt_Percentage',min([str2num(get_param(gcb,'NMC_HipFlexors_Percentage')) str2num(get_param(gcb,'NMC_HipExtensors_Percentage'))]))
      | set_param(gcb,'NMC_HipMuscles_FE_Percentage',min([str2num(get_param(gcb,'NMC_HipFlexors_Percentage')) str2num(get_param(gcb,'NMC_HipExtensors_Percentage'))]))
      | set_param(gcb,'NMC_BiArticularMuscles_HK_Percentage',min([str2num(get_param(gcb,'NMC_KneeExtensors_Percentage')) str2num(get_param(gcb,'NMC_KneeFlexors_Percentage')) str2num(get_param(gcb,'NMC_HipFlexors_Percentage')) str2num(get_param(gcb,'NMC_HipExtensors_Percentage'))]))
      | end
      mask Callback NMC_KneeFlexors_Percentage:
      | if str2num(get_param([gcb '/LimiterMethod'],'Value')) == 2;
      | %Also setting values of sliders per joint/per location
      | set_param(gcb,'NMC_KneeFlexExt_Percentage',min([str2num(get_param(gcb,'NMC_KneeExtensors_Percentage')) str2num(get_param(gcb,'NMC_KneeFlexors_Percentage'))]))
      | set_param(gcb,'NMC_KneeMuscles_Percentage',min([str2num(get_param(gcb,'NMC_KneeExtensors_Percentage')) str2num(get_param(gcb,'NMC_KneeFlexors_Percentage')) ]))
      | set_param(gcb,'NMC_BiArticularMuscles_KA_Percentage',min([str2num(get_param(gcb,'NMC_KneeFlexors_Percentage')) str2num(get_param(gcb,'NMC_AnklePFlexors_Percentage'))]))
      | set_param(gcb,'NMC_BiArticularMuscles_HK_Percentage',min([str2num(get_param(gcb,'NMC_KneeExtensors_Percentage')) str2num(get_param(gcb,'NMC_KneeFlexors_Percentage')) str2num(get_param(gcb,'NMC_HipFlexors_Percentage')) str2num(get_param(gcb,'NMC_HipExtensors_Percentage'))]))
      | end
      mask Callback NMC_KneeExtensors_Percentage:
      | if str2num(get_param([gcb '/LimiterMethod'],'Value')) == 2;
      | %Also setting values of sliders per joint/per location
      | set_param(gcb,'NMC_KneeFlexExt_Percentage',min([str2num(get_param(gcb,'NMC_KneeExtensors_Percentage')) str2num(get_param(gcb,'NMC_KneeFlexors_Percentage'))]))
      | set_param(gcb,'NMC_KneeMuscles_Percentage',min([str2num(get_param(gcb,'NMC_KneeExtensors_Percentage')) str2num(get_param(gcb,'NMC_KneeFlexors_Percentage')) ]))
      | set_param(gcb,'NMC_BiArticularMuscles_HK_Percentage',min([str2num(get_param(gcb,'NMC_KneeExtensors_Percentage')) str2num(get_param(gcb,'NMC_KneeFlexors_Percentage')) str2num(get_param(gcb,'NMC_HipFlexors_Percentage')) str2num(get_param(gcb,'NMC_HipExtensors_Percentage'))]))
      | end
      mask Callback NMC_AnkleDFlexor_Percentage:
      | if str2num(get_param([gcb '/LimiterMethod'],'Value')) == 2;
      | %Also setting values of sliders per joint/per location
      | set_param(gcb,'NMC_AnkleDorsPlant_Percentage',min([str2num(get_param(gcb,'NMC_AnklePFlexors_Percentage')) str2num(get_param(gcb,'NMC_AnkleDFlexor_Percentage'))]))
      | set_param(gcb,'NMC_AnkleMuscles_Percentage',min([str2num(get_param(gcb,'NMC_AnklePFlexors_Percentage')) str2num(get_param(gcb,'NMC_AnkleDFlexor_Percentage'))]))
      | end
      mask Callback NMC_AnklePFlexors_Percentage:
      | if str2num(get_param([gcb '/LimiterMethod'],'Value')) == 2;
      |     %Also setting values of sliders per joint/per location
      |     set_param(gcb,'NMC_AnkleDorsPlant_Percentage',min([str2num(get_param(gcb,'NMC_AnklePFlexors_Percentage')) str2num(get_param(gcb,'NMC_AnkleDFlexor_Percentage'))]))
      |     set_param(gcb,'NMC_AnkleMuscles_Percentage',min([str2num(get_param(gcb,'NMC_AnklePFlexors_Percentage')) str2num(get_param(gcb,'NMC_AnkleDFlexor_Percentage'))]))
      |     set_param(gcb,'NMC_BiArticularMuscles_KA_Percentage',min([str2num(get_param(gcb,'NMC_KneeFlexors_Percentage')) str2num(get_param(gcb,'NMC_AnklePFlexors_Percentage'))]))
      | end
      mask Callback NMC_HipMuscles_AbAd_Percentage:
      | if str2num(get_param([gcb '/LimiterMethod'],'Value')) == 3;
      |     %Also setting values of sliders per joint/per Function
      |     set_param(gcb,'NMC_HipAddAbd_Percentage',get_param(gcb,'NMC_HipMuscles_AbAd_Percentage'))
      |     set_param(gcb,'NMC_HipAdd_Percentage',get_param(gcb,'NMC_HipMuscles_AbAd_Percentage'))
      |     set_param(gcb,'NMC_HipAbd_Percentage',get_param(gcb,'NMC_HipMuscles_AbAd_Percentage'))
      | end
      mask Callback NMC_HipMuscles_FE_Percentage:
      | if str2num(get_param([gcb '/LimiterMethod'],'Value')) == 3;
      |     % Hip
      |     set_param(gcb,'NMC_HipFlexExt_Percentage',min([str2num(get_param(gcb,'NMC_HipMuscles_FE_Percentage')) str2num(get_param(gcb,'NMC_BiArticularMuscles_HK_Percentage'))]))
      |     set_param(gcb,'NMC_HipFlexors_Percentage',min([str2num(get_param(gcb,'NMC_HipMuscles_FE_Percentage')) str2num(get_param(gcb,'NMC_BiArticularMuscles_HK_Percentage'))]))
      |     set_param(gcb,'NMC_HipExtensors_Percentage',min([str2num(get_param(gcb,'NMC_HipMuscles_FE_Percentage')) str2num(get_param(gcb,'NMC_BiArticularMuscles_HK_Percentage'))]))
      | end
      mask Callback NMC_BiArticularMuscles_HK_Percentage:
      | if str2num(get_param([gcb '/LimiterMethod'],'Value')) == 3;
      |     %Also setting values of sliders per joint/per Function
      |     % Hip
      |     set_param(gcb,'NMC_HipFlexExt_Percentage',min([str2num(get_param(gcb,'NMC_HipMuscles_FE_Percentage')) str2num(get_param(gcb,'NMC_BiArticularMuscles_HK_Percentage'))]))
      |     set_param(gcb,'NMC_HipFlexors_Percentage',min([str2num(get_param(gcb,'NMC_HipMuscles_FE_Percentage')) str2num(get_param(gcb,'NMC_BiArticularMuscles_HK_Percentage'))]))
      |     set_param(gcb,'NMC_HipExtensors_Percentage',min([str2num(get_param(gcb,'NMC_HipMuscles_FE_Percentage')) str2num(get_param(gcb,'NMC_BiArticularMuscles_HK_Percentage'))]))
      |     set_param(gcb,'NMC_KneeFlexExt_Percentage',min([str2num(get_param(gcb,'NMC_KneeMuscles_Percentage')) str2num(get_param(gcb,'NMC_BiArticularMuscles_HK_Percentage')) str2num(get_param(gcb,'NMC_BiArticularMuscles_KA_Percentage'))]))
      |     set_param(gcb,'NMC_KneeFlexors_Percentage',min([str2num(get_param(gcb,'NMC_KneeMuscles_Percentage')) str2num(get_param(gcb,'NMC_BiArticularMuscles_HK_Percentage')) str2num(get_param(gcb,'NMC_BiArticularMuscles_KA_Percentage'))]))
      |     set_param(gcb,'NMC_KneeExtensors_Percentage',min([str2num(get_param(gcb,'NMC_KneeMuscles_Percentage')) str2num(get_param(gcb,'NMC_BiArticularMuscles_HK_Percentage'))]))
      | end
      mask Callback NMC_KneeMuscles_Percentage:
      | if str2num(get_param([gcb '/LimiterMethod'],'Value')) == 3;
      |     % Knee
      |     set_param(gcb,'NMC_KneeFlexExt_Percentage',min([str2num(get_param(gcb,'NMC_KneeMuscles_Percentage')) str2num(get_param(gcb,'NMC_BiArticularMuscles_HK_Percentage')) str2num(get_param(gcb,'NMC_BiArticularMuscles_KA_Percentage'))]))
      |     set_param(gcb,'NMC_KneeFlexors_Percentage',min([str2num(get_param(gcb,'NMC_KneeMuscles_Percentage')) str2num(get_param(gcb,'NMC_BiArticularMuscles_HK_Percentage')) str2num(get_param(gcb,'NMC_BiArticularMuscles_KA_Percentage'))]))
      |     set_param(gcb,'NMC_KneeExtensors_Percentage',min([str2num(get_param(gcb,'NMC_KneeMuscles_Percentage')) str2num(get_param(gcb,'NMC_BiArticularMuscles_HK_Percentage'))]))
      | end
      mask Callback NMC_BiArticularMuscles_KA_Percentage:
      | if str2num(get_param([gcb '/LimiterMethod'],'Value')) == 3;
      |     % Ankle
      |     set_param(gcb,'NMC_AnkleDorsPlant_Percentage',min([str2num(get_param(gcb,'NMC_AnkleMuscles_Percentage')) str2num(get_param(gcb,'NMC_BiArticularMuscles_KA_Percentage'))]))
      |     set_param(gcb,'NMC_AnklePFlexors_Percentage',min([str2num(get_param(gcb,'NMC_AnkleMuscles_Percentage')) str2num(get_param(gcb,'NMC_BiArticularMuscles_KA_Percentage'))]))
      |     set_param(gcb,'NMC_KneeFlexExt_Percentage',min([str2num(get_param(gcb,'NMC_KneeMuscles_Percentage')) str2num(get_param(gcb,'NMC_BiArticularMuscles_HK_Percentage')) str2num(get_param(gcb,'NMC_BiArticularMuscles_KA_Percentage'))]))
      |     set_param(gcb,'NMC_KneeFlexors_Percentage',min([str2num(get_param(gcb,'NMC_KneeMuscles_Percentage')) str2num(get_param(gcb,'NMC_BiArticularMuscles_HK_Percentage')) str2num(get_param(gcb,'NMC_BiArticularMuscles_KA_Percentage'))]))
      | end
      mask Callback NMC_AnkleMuscles_Percentage:
      | if str2num(get_param([gcb '/LimiterMethod'],'Value')) == 3;
      |     % Ankle
      |     set_param(gcb,'NMC_AnkleDorsPlant_Percentage',min([str2num(get_param(gcb,'NMC_AnkleMuscles_Percentage')) str2num(get_param(gcb,'NMC_BiArticularMuscles_KA_Percentage'))]))
      |     set_param(gcb,'NMC_AnkleDFlexor_Percentage',min([str2num(get_param(gcb,'NMC_AnkleMuscles_Percentage'))]))
      |     set_param(gcb,'NMC_AnklePFlexors_Percentage',min([str2num(get_param(gcb,'NMC_AnkleMuscles_Percentage')) str2num(get_param(gcb,'NMC_BiArticularMuscles_KA_Percentage'))]))
      | end
      mask TypeOptions EnableJointLimits: Enable | Disable
      mask Callback EnableJointLimits:
      | button_value = get_param(gcb,'EnableJointLimits');
      | 
      | if strcmp(button_value,'Enable')
      |      set_param([gcb '/EnableJointLimits'],'Value',num2str(1));
      | else
      |     set_param([gcb '/EnableJointLimits'],'Value',num2str(0));
      | end
      mask TypeOptions UseConstantPitch: Enable | Disable
      mask Callback UseConstantPitch:
      | button_value = get_param(gcb,'UseConstantPitch');
      | 
      | if strcmp(button_value,'Enable')
      |      set_param([gcb '/UseConstantPitch'],'Value',num2str(1));
      | else
      |     set_param([gcb '/UseConstantPitch'],'Value',num2str(0));
      | end
      mask TypeOptions UsePredictedAnkle: Enable | Disable
      mask Callback UsePredictedAnkle:
      | button_value = get_param(gcb,'UsePredictedAnkle');
      | 
      | if strcmp(button_value,'Enable')
      |      set_param([gcb '/UsePredictedAnkle'],'Value',num2str(1));
      | else
      |     set_param([gcb '/UsePredictedAnkle'],'Value',num2str(0));
      | end
      mask TypeOptions EnableStandingStill: Enable | Disable
      mask Callback EnableStandingStill:
      | button_value = get_param(gcb,'EnableStandingStill');
      | 
      | if strcmp(button_value,'Enable')
      |      set_param([gcb '/EnableStandingStill'],'Value',num2str(1));
      | else
      |     set_param([gcb '/EnableStandingStill'],'Value',num2str(0));
      | end
      mask DialogControl Control2 Prompt: LOPES Info
      mask DialogControl Control3 Prompt: Refresh
      mask DialogControl Control3 Callback:
      | rto = get_param([gcb,'/LopesStateShow'], 'RunTimeObject');
      | if isempty(rto)
      |     set_param(gcb,'InfoShow_LLC','Not Connected')
      |     set_param(gcb,'InfoShow_Blue','Not Connected')
      |     set_param(gcb,'InfoShow_Init','Not Connected')
      |     set_param(gcb,'InfoShow_Motors','Not Connected')
      |     set_param(gcb,'InfoShow_Treadmill','Not Connected')
      |     set_param(gcb,'InfoShow_Patient','Not Connected')
      | else
      |     p = get(rto.InputPort(1));values = p.Data;
      |     set_param(gcb,'InfoShow_LLC',num2str(values(1)))
      |     set_param(gcb,'InfoShow_Blue',num2str(values(2)))
      |     set_param(gcb,'InfoShow_Init',num2str(values(3)))
      |     set_param(gcb,'InfoShow_Motors',num2str(values(4)))
      |     set_param(gcb,'InfoShow_Treadmill',num2str(values(5)))
      |     set_param(gcb,'InfoShow_Patient',num2str(values(6)))
      | end
      mask DialogControl Container34 Prompt: POS Main Settings
      mask DialogControl Container21_copy Prompt: General Gains
      mask DialogControl Container21 Prompt: General Gains
      mask DialogControl Container22 Prompt: Limiters
      mask DialogControl DescTextVar Prompt: Per Joint/Per Function/Per Gradient:
      mask DialogControl ParameterGroupVar_copy Prompt: Slide to Adjust:
      mask DialogControl ParameterGroupVar Prompt: Slide to Adjust:
      mask DialogControl Container11 Prompt: Slide To Adjust
      mask DialogControl Container50 Prompt: Standing Still:
  NMC Model : nmc/NMC Model
  NMC_Control : Concatenate  NumInputs=1
  NMC_Limiters : Concatenate  NumInputs=1
  NMC_TorqueController : Concatenate  NumInputs=1
  NMC_TorquePure : Concatenate  NumInputs=1
  OveralGainLabel : nmc/OveralGainLabel
  Pos/NMCGain : ManualSwitch
  PosSwitchSettings : Concatenate  NumInputs=1
  Product{,1,4..5} (4 alike) : Product
  RL_enable : nmc/RL_enable
  RL_enable3 : nmc/RL_enable
  Right{,1,5..6} (4 alike) : Selector  InputPortWidth=SelectorScopesSize  IndexOptions=Index vector (dialog)  Indices=SelectorScopesRight  OutputSizes=1
  Right2 : Selector  InputPortWidth=8  IndexOptions=Index vector (dialog)  Indices=[1,2,3,4]  OutputSizes=1
  Right3 : Selector  Commented=on  InputPortWidth=SelectorScopesSize  IndexOptions=Index vector (dialog)  Indices=SelectorScopesRight  OutputSizes=1
  Right4 : Selector  Commented=on  InputPortWidth=SelectorScopesSize  IndexOptions=Index vector (dialog)  Indices=SelectorScopesRight  OutputSizes=1
  RightAngles : Selector  InputPortWidth=16  IndexOptions=Index vector (dialog)  Indices=[9,11,13,15]  OutputSizes=1
  RightAnglesPos : Selector  InputPortWidth=SelectorLOPESModelPosSize  IndexOptions=Index vector (dialog)  Indices=SelectorScopesRight  OutputSizes=1
  SaveSwitch : Subsystem
  "Scope (xPC) " : slrtlib/Displays and Logging/Scope   scopeno=1  scopetype=File  autostart=on  viewmode=Graphical redraw  formatstr='%15.6f'  grid=on  ylimits=[0,0]  nosamples=250  noprepostsamples=0  interleave=1  triggermode=FreeRun  triggersignal=1  trigsignalfromport=off  triggerlevel=0.0  triggerslope=Either  triggerscope=1  triggersample=0  filename=data.dat  mode=Lazy  writesize=512  autorestart=on  dynamicfilemode=off  maxwritefilesize=512*1024^2
  Scope 1 : slrtlib/Displays and Logging/Scope   scopeno=2  scopetype=Target  autostart=on  viewmode=Graphical sliding  formatstr='%15.6f'  grid=on  ylimits=[0,0]  nosamples=5000  noprepostsamples=0  interleave=1  triggermode=FreeRun  triggersignal=1  trigsignalfromport=off  triggerlevel=0.0  triggerslope=Either  triggerscope=1  triggersample=0  filename=data.dat  mode=Lazy  writesize=512  autorestart=off  dynamicfilemode=off  maxwritefilesize=512*1024^2
  Scope 2 : slrtlib/Displays and Logging/Scope   scopeno=3  scopetype=Target  autostart=on  viewmode=Graphical sliding  formatstr='%15.6f'  grid=on  ylimits=[0,0]  nosamples=5000  noprepostsamples=0  interleave=1  triggermode=FreeRun  triggersignal=1  trigsignalfromport=off  triggerlevel=0.0  triggerslope=Either  triggerscope=1  triggersample=0  filename=data.dat  mode=Lazy  writesize=512  autorestart=off  dynamicfilemode=off  maxwritefilesize=512*1024^2
  Scope 3 : slrtlib/Displays and Logging/Scope   scopeno=5  scopetype=Target  autostart=on  viewmode=Graphical sliding  formatstr='%15.6f'  grid=on  ylimits=[0,0]  nosamples=5000  noprepostsamples=0  interleave=1  triggermode=FreeRun  triggersignal=1  trigsignalfromport=off  triggerlevel=0.0  triggerslope=Either  triggerscope=1  triggersample=0  filename=data.dat  mode=Lazy  writesize=512  autorestart=off  dynamicfilemode=off  maxwritefilesize=512*1024^2
  Scope 4 : slrtlib/Displays and Logging/Scope   scopeno=4  scopetype=Target  autostart=on  viewmode=Graphical sliding  formatstr='%15.6f'  grid=on  ylimits=[0,0]  nosamples=5000  noprepostsamples=0  interleave=1  triggermode=FreeRun  triggersignal=1  trigsignalfromport=off  triggerlevel=0.0  triggerslope=Either  triggerscope=1  triggersample=0  filename=data.dat  mode=Lazy  writesize=512  autorestart=off  dynamicfilemode=off  maxwritefilesize=512*1024^2
  Scope 5 : slrtlib/Displays and Logging/Scope   Commented=on  scopeno=2  scopetype=Target  autostart=on  viewmode=Graphical sliding  formatstr='%15.6f'  grid=on  ylimits=[0,0]  nosamples=5000  noprepostsamples=0  interleave=1  triggermode=FreeRun  triggersignal=1  trigsignalfromport=off  triggerlevel=0.0  triggerslope=Either  triggerscope=1  triggersample=0  filename=data.dat  mode=Lazy  writesize=512  autorestart=off  dynamicfilemode=off  maxwritefilesize=512*1024^2
  Scope 6 : slrtlib/Displays and Logging/Scope   scopeno=10  scopetype=Target  autostart=on  viewmode=Graphical sliding  formatstr='%15.6f'  grid=on  ylimits=[-0.1,1]  nosamples=5000  noprepostsamples=0  interleave=1  triggermode=FreeRun  triggersignal=1  trigsignalfromport=off  triggerlevel=0.0  triggerslope=Either  triggerscope=1  triggersample=0  filename=data.dat  mode=Lazy  writesize=512  autorestart=off  dynamicfilemode=off  maxwritefilesize=512*1024^2
  Selector1 : Selector  InputPortWidth=7  IndexOptions=Index vector (dialog)  Indices=[2]  OutputSizes=1
  Selector3 : Selector  Commented=on  InputPortWidth=7  IndexOptions=Index vector (dialog)  Indices=[2]  OutputSizes=1
  Selector5 : Selector  InputPortWidth=SelectorLOPESModelPosSize  IndexOptions=Index vector (dialog)  Indices=SelectActive  OutputSizes=1
  Selector6 : Selector  InputPortWidth=10  IndexOptions=Index vector (dialog)  Indices=SelectorLOPESIn  OutputSizes=1
  Settings : Subsystem
  Simple Linear Switch : Subsystem
  StateDiagram : Stateflow chart
      settings: MinAlgLoopOccurrences=on
  Terminator1 : Terminator
  Terminator3 : Terminator
  ToLopes : LopesDevelopmentLibrary/Robot control blocks/ToLopes
  ToLopes_SpringPositions : Concatenate  NumInputs=1
  ToLopes_SpringStiffness : Concatenate  NumInputs=1
  TorqueLimiter : Subsystem
  Tunnel Switch : Subsystem
  Up/Down : ManualSwitch  CurrentSetting=0
  Up/Down1 : ManualSwitch  CurrentSetting=0
  Up/Down2 : ManualSwitch  Commented=on  CurrentSetting=0
  Up/Down3 : ManualSwitch  Commented=on
  VelocityHold : LopesDevelopmentLibrary/GaitGenerationExtra/VelocityHold
  cst : Constant  Value=0
  wAnkleConvert : Selector  InputPortWidth=SelectorCartPosSize  IndexOptions=Index vector (dialog)  Indices=SelectorCartPos  OutputSizes=1
  tag scope: EstimatedPhase=global, LopesLLCState=global, LopesState=global, NMCBiasForceGain=global, PhaseIn=global, PosSpringGain=global
  wires:
  FromLopes/1 -> ErrorFromLopes/1
  [LopesDesiredState] -> GeneralLopes/1
  GeneralLopes/1 -> Error/1
  GeneralLopes/2 -> [LopesState], ToLopes/1, Bus Selector/1
  ToLopes/1 -> ErrorToLopes/1
  FromLopes/3 -> [LopesModelVel]
  FromLopes/4 -> Terminator1/1
  FromLopes/6 -> [LopesMeasForces]
  FromLopes/8 -> Gait Phase Detection with Wrapper/2, [LopesTreadmill]
  EnableEffects/1 -> ToLopes/8
  [TreadmillVelocityOut] -> ToLopes/7
  ToLopes/2 -> EffectsFullyEnabled/1
  FromLopes/2 -> [LopesModelPos]
  [LopesModelPos] -> ToLopes/2
  cst/1 -> Mux/1, Mux/2
  FromLopes/5 -> Terminator3/1
  [PhaseIn] -> FromLOPES_StanceDetection/1
  FromLOPES_StanceDetection/1 -> Mux2/1
  [LopesModelPos] -> FromLOPES_MeasPos/1
  FromLOPES_MeasPos/1 -> Mux2/2
  [LopesCartesianPositionsFull] -> FromLOPES_CartesianPositions/1
  FromLOPES_CartesianPositions/1 -> Mux2/4
  [LopesModelVel] -> FromLOPES_ModelVel/1
  FromLOPES_ModelVel/1 -> Mux2/3
  [LopesTreadmill] -> FromLOPES_Treadmill/1
  FromLOPES_Treadmill/1 -> Mux2/5
  [SpringPositionsOut] -> ToLopes/3
  [SpringStiffness] -> ToLopes/5
  FromLopes/9 -> AnalogInput9_16/1
  Mux/1 -> Product4/1
  Mux2/1 -> "Scope (xPC) "/1
  Bus Selector/1 -> [LopesLLCState]  "<llcState>"
  Mux3/1 -> [TorqueFromNMC]
  [LopesTreadmill] -> Selector1/1
  Selector1/1 -> Mux4/1  "Velocity"
  [PhaseIn] -> Gain5/1
  Gain5/1 -> Mux4/2  "Phase"
  Mux4/1 -> LabelPhase/1(Sigs)
  [LopesModelPos] -> LeftAnglesPos/1, RightAnglesPos/1
  Gait Phase Detection with Wrapper/1 -> [PhaseIn]
  Product4/1 -> Selector6/1
  [OverallPosEnable] -> Pos/NMCGain/1  "PosGain"
  [OverallNMCEnable] -> Pos/NMCGain/2  "NMCGain"
  NMC Model/8 -> Mux3/8, TorqueLimiter/8(In8)
  NMC Model/7 -> Mux3/7, TorqueLimiter/7(In7)
  NMC Model/4 -> Mux3/4, TorqueLimiter/4(In6)
  NMC Model/3 -> Mux3/3, TorqueLimiter/3(In5)
  [LopesMeasForces] -> FromLopes_MeasForces/1
  FromLopes_MeasForces/1 -> Mux2/6
  NMC Model/1 -> Mux3/1, TorqueLimiter/1(In1)
  NMC Model/5 -> Mux3/5, TorqueLimiter/5(In3)
  [LopesControllerOut] -> ToLopes/6
  [LopesCartesianPositions] -> LopesToGeyer_cart/1
  LopesToGeyer_cart/1 -> Mux1/1
  LopesToGeyer_cart/9 -> Mux1/9
  LopesToGeyer_cart/7 -> Mux1/7
  LopesToGeyer_cart/10 -> Mux1/10
  LopesToGeyer_cart/4 -> Mux1/4
  LopesToGeyer_cart/2 -> Mux1/2
  LopesToGeyer_cart/5 -> Mux1/5
  LopesToGeyer_cart/3 -> Mux1/3
  LopesToGeyer_cart/6 -> Mux1/6
  LopesToGeyer_cart/8 -> Mux1/8
  Mux1/1 -> NMC Model/2
  [LopesCartesianPositions] -> LopesToGeyer_loads/1
  [LopesTreadmill] -> LopesToGeyer_loads/2
  LopesToGeyer_loads/1 -> Mux7/1
  LopesToGeyer_loads/2 -> Mux7/2
  Mux7/1 -> NMC Model/3
  [PhaseIn] -> NMC Model/5
  Compare To Constant/1 -> NMC Model/Enable
  Settings/1(Settings) -> NMC Model/4
  NMC Model/2 -> Mux3/2, TorqueLimiter/2(In2)
  NMC Model/6 -> Mux3/6, TorqueLimiter/6(In4)
  Up/Down1/1 -> LabelTorque/1(In1)
  Hip Abd/Flex1/1 -> Up/Down1/1
  [TorqueFromNMC] -> Left2/1, Right2/1
  Demux/1 -> Hip Abd/Flex1/1
  Demux/2 -> Hip Abd/Flex1/2
  [LopesLLCState] -> Compare To Constant/1
  Demux/3 -> Knee/Ankle1/1
  Demux/4 -> Knee/Ankle1/2
  Knee/Ankle1/1 -> Up/Down1/2
  Lopes LLC State/1 -> Mux2/7
  [LopesLLCState] -> Lopes LLC State/1
  [SpringPositionsOut] -> ToLopes_SpringPositions/1
  ToLopes_SpringPositions/1 -> Mux2/9
  [SpringStiffness] -> ToLopes_SpringStiffness/1
  ToLopes_SpringStiffness/1 -> Mux2/10
  [PosSwitchSettings] -> PosSwitchSettings/1
  PosSwitchSettings/1 -> Mux2/8
  HipFl/HipAb/1 -> Up/Down/1
  Demux1/1 -> HipFl/HipAb/1
  Demux1/2 -> HipFl/HipAb/2
  Demux1/3 -> Knee/Ankle/1
  Demux1/4 -> Knee/Ankle/2
  Knee/Ankle/1 -> Up/Down/2
  [GeyerAngles] -> RightAngles/1, LeftAngles/1
  Up/Down/1 -> LabelAngles/1(In1)
  [NMCMainControl] -> NMC_Control/1
  NMC_TorquePure/1 -> Mux2/12
  [LopesControllerOut] -> NMC_TorqueController/1
  NMC_TorqueController/1 -> Mux2/13
  NMC_Control/1 -> Mux2/11
  [TorqueFromNMC] -> NMC_TorquePure/1
  [LHipTau] -> Mux/4
  [RKneeTau] -> Mux/9
  [RHipTauRoll] -> Mux/7
  Left/Right/1 -> Demux1/1
  RightAngles/1 -> Left/Right/2
  LeftAngles/1 -> Left/Right/1
  [EstimatedPhase] -> Gain4/1
  Gain4/1 -> Mux4/3
  Left/Right2/1 -> Demux/1
  Left2/1 -> Left/Right2/1
  Right2/1 -> Left/Right2/2
  LabelPhase/1(LabSigs) -> Scope 1/1
  TorqueLimiter/1(Out1) -> Filter/1(In1)
  TorqueLimiter/5(Out3) -> Filter/5(In3)
  TorqueLimiter/8(Out8) -> Filter/8(In8)
  TorqueLimiter/7(Out7) -> Filter/7(In7)
  TorqueLimiter/6(Out4) -> Filter/6(In4)
  TorqueLimiter/4(Out6) -> Filter/4(In6)
  TorqueLimiter/3(Out5) -> Filter/3(In5)
  TorqueLimiter/2(Out2) -> Filter/2(In2)
  Filter/1(Out1) -> [RHipTau]
  Filter/2(Out2) -> [RHipTauRoll]
  Filter/3(Out5) -> [RKneeTau]
  Filter/4(Out6) -> [RAnkleTau]
  Filter/5(Out3) -> [LHipTau]
  Filter/6(Out4) -> [LHipTauRoll]
  Filter/7(Out7) -> [LKneeTau]
  Filter/8(Out8) -> [LAnkleTau]
  [RHipTau] -> Mux/8
  [RAnkleTau] -> Mux/10
  [LAnkleTau] -> Mux/6
  [LKneeTau] -> Mux/5
  [LHipTauRoll] -> Mux/3
  [EnableNMC] -> RL_enable/1
  Product1/1 -> [LopesControllerOut]
  [LopesControllerOut] -> Left/1, Right/1
  Left/1 -> Left/Right1/1
  Right/1 -> Left/Right1/2
  FromLopes/7 -> [LopesCartesianPositionsFull], Gait Phase Detection with Wrapper/1, wAnkleConvert/1
  [LopesModelPos] -> LopesToGeyer_angles/1
  [LopesModelVel] -> LopesToGeyer_angles/2
  LopesToGeyer_angles/3 -> Mux6/3
  LopesToGeyer_angles/4 -> Mux6/4
  LopesToGeyer_angles/1 -> Mux6/1
  LopesToGeyer_angles/5 -> Mux6/5
  LopesToGeyer_angles/6 -> Mux6/6
  LopesToGeyer_angles/7 -> Mux6/7
  LopesToGeyer_angles/2 -> Mux6/2
  LopesToGeyer_angles/8 -> Mux6/8
  Mux6/1 -> NMC Model/1, [GeyerAngles]
  Left/Right1/1 -> LopesTorqueOutLabel/1
  [SpringPositions] -> Left1/1, Right1/1
  Left1/1 -> Left/Right3/1
  Right1/1 -> Left/Right3/2
  Left/Right3/1 -> LopesSpringPosLabel/1
  From62/1 -> Selector3/1
  Selector3/1 -> Mux9/1  "Velocity"
  From64/1 -> Gain2/1
  Gain2/1 -> Mux9/2  "Phase"
  Mux9/1 -> Label1/1(In1)
  From67/1 -> Gain1/1
  Gain1/1 -> Mux9/3
  Label1/1(Out1) -> Scope 5/1
  Mux5/1 -> Label4/1(In1)
  From26/1 -> Mux5/1  "PosGain"
  From10/1 -> Mux5/2  "NMCGain"
  Label4/1(Out1) -> Forces6/1
  From68/1 -> Left3/1, Right3/1
  Left3/1 -> Left/Right4/1
  Right3/1 -> Left/Right4/2
  Mux10/1 -> Label6/1(In1)
  From69/1 -> Gain/1
  Gain/1 -> Mux10/2
  Up/Down2/1 -> Mux10/1
  Hip Abd/Flex2/1 -> Up/Down2/1
  Demux2/1 -> Hip Abd/Flex2/1
  Demux2/2 -> Hip Abd/Flex2/2
  Demux2/3 -> Up/Down2/2
  Left/Right4/1 -> Demux2/1
  From70/1 -> Left4/1, Right4/1
  Left4/1 -> Left/Right5/1
  Right4/1 -> Left/Right5/2
  Hip Abd/Flex3/1 -> Up/Down3/1
  Demux3/1 -> Hip Abd/Flex3/1
  Demux3/2 -> Hip Abd/Flex3/2
  Demux3/3 -> Up/Down3/2
  Left/Right5/1 -> Demux3/1
  Up/Down3/1 -> Mux11/1
  Mux11/1 -> Label5/1(In1)
  From71/1 -> Gain3/1
  Gain3/1 -> Mux11/2
  Label5/1(Out1) -> Forces7/1
  Label6/1(Out1) -> Forces5/1
  Product/1 -> [OverallNMCEnable]
  [LopesTreadmill] -> LopesToGeyer_cart/2
  [AnalogInput] -> AnalogInput/1
  AnalogInput/1 -> Mux2/14
  AnalogInput9_16/1 -> [AnalogInput]
  [AnalogInput] -> FilterEMG/1(In1)
  FilterEMG/1(Out1) -> Gain6/1
  [SpringVelocities] -> ToLopes/4
  [NMCBiasForceGain] -> Product/1, Product1/2
  Selector6/1 -> Product1/1
  RL_enable/1 -> Product/2, Product4/2
  [TunnelStop] -> Tunnel Switch/2(TunnelEnd)
  [TunnelStart] -> Tunnel Switch/1(TunnelStart)
  Selector5/1 -> Tunnel Switch/3(CurAngles)
  [SpringPositions] -> Tunnel Switch/4(RefAngles)
  [LopesModelPos] -> Selector5/1
  Tunnel Switch/3(TunnelOffset) -> SaveSwitch/7("TunnelOffset ")
  Simple Linear Switch/1(pos_gain) -> SaveSwitch/3(PosGainLin)
  Tunnel Switch/1(pos_gain) -> SaveSwitch/5(PosGainTunnel)
  Simple Linear Switch/2(NMC_gain) -> SaveSwitch/4(NMCGainLin)
  Tunnel Switch/2(NMC_gain) -> SaveSwitch/6(NMCGainTunnel)
  [SpringPositions] -> SaveSwitch/2(PosSpring)
  SaveSwitch/1(PosGain) -> [PosSpringGain]
  SaveSwitch/3(NMCGain) -> [NMCBiasForceGain]
  SaveSwitch/2(SpringPosOut) -> [SpringPositionsOut]
  [TorqueLimiters] -> NMC_Limiters/1
  NMC_Limiters/1 -> Mux2/15
  Gain6/1 -> LabelEMG/1(Sigs)
  LabelEMG/1(LabSigs) -> Scope 6/1
  [LopesModelPos] -> GaitGenerationAndAnalysis/1
  [LopesModelVel] -> GaitGenerationAndAnalysis/2
  GaitGenerationAndAnalysis/4 -> [EstimatedPhase]
  GaitGenerationAndAnalysis/3 -> [SpringStiffness]
  GaitGenerationAndAnalysis/2 -> [SpringVelocities]
  [EnablePos] -> RL_enable3/1
  RL_enable3/1 -> Math Function3/1
  Math Function3/1 -> Product5/1
  Product5/1 -> [OverallPosEnable]
  [PosSpringGain] -> Product5/2
  GaitGenerationAndAnalysis/1 -> [SpringPositions]
  wAnkleConvert/1 -> [LopesCartesianPositions]
  GaitGenerationAndAnalysis/5 -> [TreadmillVelocityOut]
  StateDiagram/1(State) -> Display2/1, VelocityHold/1, GaitGenerationAndAnalysis/3
  [StateDiagram_InputState] -> StateDiagram/1(InputState)
  [EstimatedPhase] -> StateDiagram/2(PhasePerc)
  [PhaseIn] -> StateDiagram/3(MeasPhase)
  [StateDiagram_StartLeg] -> StateDiagram/4(StartLeg)
  "1 = Left, 2 = right"/1 -> [StateDiagram_StartLeg]
  VelocityHold/1 -> GaitGenerationAndAnalysis/4
  [LopesTreadmill] -> GetInputStateFromVelocity/1(RealVelocity)
  [TreadmillVelocityIn] -> GetInputStateFromVelocity/2(DesVelocity)
  GetInputStateFromVelocity/1(State) -> [StateDiagram_InputState]
  [StateDiagram_InputState] -> VelocityHold/2
  [TreadmillVelocityIn] -> VelocityHold/3
  [SwitchMethod] -> SaveSwitch/1(SwitchMethod)
  RightAnglesPos/1 -> Left/Right6/2
  LeftAnglesPos/1 -> Left/Right6/1  "LopesModelPos"
  Left/Right6/1 -> LopesModelPosLabel/1
  LabelAngles/1(Out1) -> Scope 3/1
  LabelTorque/1(Out1) -> Forces2/1
  LopesModelPosLabel/1 -> Scope 2/1
  LopesSpringPosLabel/1 -> Scope 4/1
  [LopesMeasForces] -> Left5/1, Right5/1
  Left5/1 -> Left/Right7/1
  Right5/1 -> Left/Right7/2
  Left/Right7/1 -> LopesMeasForceLabel/1
  LopesMeasForceLabel/1 -> Forces/1
  Pos/NMCGain/1 -> Right6/1, Left6/1
  Left6/1 -> "Left/Right8 "/1
  Right6/1 -> "Left/Right8 "/2
  "Left/Right8 "/1 -> OveralGainLabel/1
  OveralGainLabel/1 -> Forces1/1
  LopesTorqueOutLabel/1 -> Forces4/1
  [LopesTreadmill] -> CurrentVelocity/1
  CurrentVelocity/1 -> NMC Model/6
  [LopesLLCState] -> Compare To Constant1/1
  Compare To Constant1/1 -> GetInputStateFromVelocity/3(LopesState)
  [LopesLLCState] -> VelocityHold/4
